simulink model "PositionTransitionHandler"  (R2016b)
settings: Solver=FixedStepAuto  StartTime=0.0  StopTime=10.0  RelTol=1e-3  EnableMultiTasking=on
settings Model: Creator=march  LastModifiedBy=march
settings SolverCC: EnableConcurrentExecution=on
settings DataIOCC: SaveFormat=StructureWithTime
settings OptimizationCC: BlockReduction=off  OptimizeBlockIOStorage=off  BufferReuse=off  GlobalBufferReuse=off  ExpressionFolding=off  LocalBlockOutputs=off
settings HardwareCC: ProdBitPerPointer=32  ProdBitPerSizeT=32  ProdBitPerPtrDiffT=32  ProdLargestAtomicFloat=None  ProdWordSize=32  ProdLongLongMode=on  ProdHWDeviceType=Generic->32-bit x86 compatible
settings RTWCC: SystemTargetFile=slrt.tlc  TemplateMakefile=slrt_default_tmf  Description=Simulink Real-Time  RTWCompilerOptimization=on

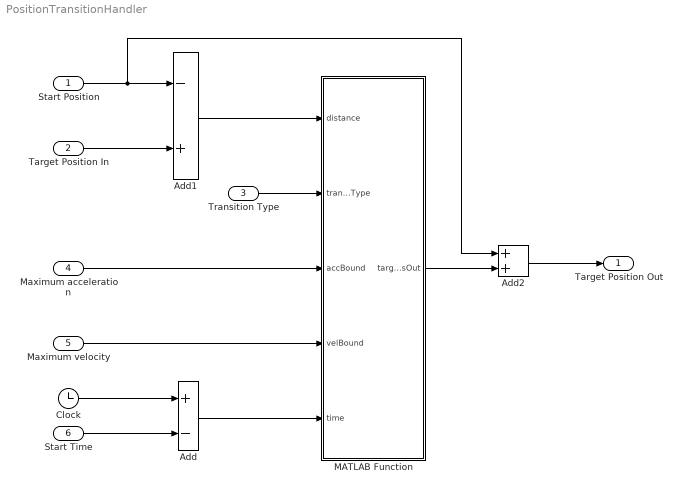
== system PositionTransitionHandler ==
  Start Position : Inport
  Target Position In : Inport  Port=2
  Transition Type : Inport  Port=3
  Maximum acceleration : Inport  Port=4
  Maximum velocity : Inport  Port=5
  Start Time : Inport  Port=6
  Add : Sum  Inputs=+-
  Add1 : Sum  Inputs=-+
  Add2 : Sum
  Clock : Clock
  MATLAB Function : MATLAB Function  TreatAsAtomicUnit=on
  Target Position Out : Outport
  wires:
  Clock/1 -> Add/1
  Start Time/1 -> Add/2
  Target Position In/1 -> Add1/2
  Start Position/1 -> Add2/1, Add1/1
  Add1/1 -> MATLAB Function/1(distance)
  Transition Type/1 -> MATLAB Function/2(transitionType)
  Maximum acceleration/1 -> MATLAB Function/3(accBound)
  Maximum velocity/1 -> MATLAB Function/4(velBound)
  Add/1 -> MATLAB Function/5(time)
  MATLAB Function/1(targetPosOut) -> Add2/2
  Add2/1 -> Target Position Out/1

== matlab function PositionTransitionHandler/MATLAB Function ==
  data: distance input; targetPosOut output; transitionType input; accBound input; velBound input; time input
function targetPosOut = getTargetPosOut(distance, transitionType, accBound, velBound, time)
timeNeeded = 2*sqrt(abs(distance)/accBound);
maxVel = accBound*timeNeeded/2;
if maxVel >= velBound % then we need three parts
    timeNeeded = abs(distance)/velBound + velBound/accBound;
    timeToStopAcc = velBound/accBound;
    timeToStartDec = timeNeeded - timeToStopAcc;
    if time < timeToStopAcc
        curTargetVel = accBound * time * sign(distance);
        targetPosOut = 0.5 * curTargetVel * time;
    elseif time > timeToStartDec
        curTargetVel = (velBound - accBound * (time - timeToStartDec));
        travelledPos = (0.5 * velBound * timeToStopAcc + (timeNeeded - 2*timeToStopAcc)*velBound);
        targetPosOut = (travelledPos + (0.5 * velBound * timeToStopAcc - 0.5 * curTargetVel * (timeNeeded - time)))*sign(distance);
    else
        travelledPos = 0.5 * velBound * timeToStopAcc;
        targetPosOut = (travelledPos + velBound * (time- timeToStopAcc))*sign(distance);
    end
else
    midTime = timeNeeded/2;
    maxSpeed = accBound * midTime;
    if time < midTime
        curTargetVel = accBound * time;
        targetPosOut = (0.5 * curTargetVel * time)*sign(distance);
    else
        travelledPos = 0.5 * maxSpeed * midTime;
        curTargetVel = maxSpeed - accBound * (time - midTime);
        targetPosOut = (travelledPos + (0.5 * maxSpeed * midTime - 0.5 * curTargetVel * (timeNeeded - time)))*sign(distance);
    end
end
if time > timeNeeded
    targetPosOut = distance;
end
end
